simulink model "Events3"  (Simulink 5.0)
settings: Solver=ode45  StartTime=0.0  StopTime=10.0  RelTol=1e-3
settings Model: Creator=scaife  LastModifiedBy=scaife  ExtModeAutoUpdateStatusClock=off

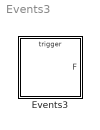
== system Events3 ==
  Events3 : Stateflow chart

== stateflow chart Events3 ==
  state TOP1 [parallel]
    state A
    state B
    (default) -> A
    A -> B : G/E;
    B -> A : G/E;
  state TOP2 [parallel]
    state C
    state D
    (default) -> C
    C -> D : E/F;
    D -> C : E/F;
  events: E local EITHER_EDGE_EVENT; F output EITHER_EDGE_EVENT; G input RISING_EDGE_EVENT
